simulink model "Simulink_UDP"  (R2022a)
settings: Solver=FixedStepAuto  StartTime=0.0  StopTime=100  FixedStep=0.001  RelTol=1e-3
libraries: dspnetwork x2
settings Model: Creator=dongxh  LastModifiedBy=dongxh

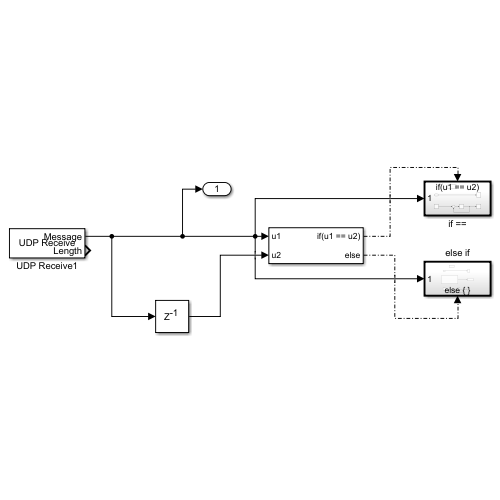
[thumbnail: Simulink's stored preview of the top-level diagram]
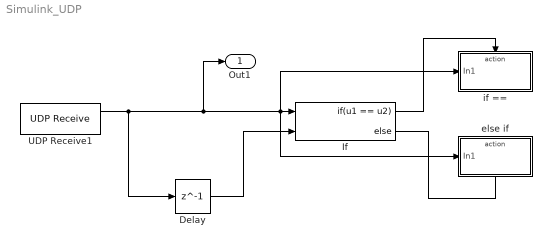
== system Simulink_UDP ==
  Delay : Delay  DelayLength=1  InitialCondition=0
  If : If  NumInputs=2  IfExpression=u1 == u2
  UDP Receive1 : dspnetwork/UDP Receive  localURL='0.0.0.0'  localPort=8002  remoteURL='127.0.0.1'  remotePort=-1  recvBufferSize=16  dims=1  signalDatatype=double  isComplex=off  isVarSize=off  showBlockingTime=off  blockingTime=0  sampletime=0.001  blockPlatform=[]
  else if : Subsystem  TreatAsAtomicUnit=on
  if == : Subsystem  TreatAsAtomicUnit=on
  Out1 : Outport
  wires:
  UDP Receive1/1 -> Delay/1, Out1/1, if ==/1(In1), If/1, else if/1(In1)
  Delay/1 -> If/2
  If/1 -> if ==/Action
  If/2 -> else if/Action

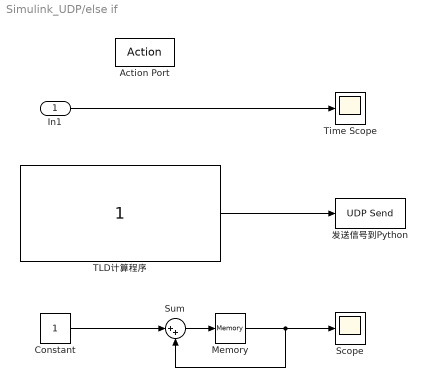
== system Simulink_UDP/else if ==
  In1 : Inport
  Action Port : ActionPort  ActionPortLabel=else
  Constant : Constant
  Memory : Memory  InheritSampleTime=on
  Scope : Scope
  Sum : Sum  Inputs=|++
  TLD计算程序 : Constant
  Time Scope : Scope
  发送信号到Python : dspnetwork/UDP Send  remoteURL='127.0.0.1'  remotePort=8004  localURL='0.0.0.0'  localPortSource=Specify via dialog  localPort=8001  sendBufferSize=16  sampletime=-1  blockPlatform=[]  separateLengthPort=0
  wires:
  Constant/1 -> Sum/1
  Sum/1 -> Memory/1
  Memory/1 -> Sum/2, Scope/1
  In1/1 -> Time Scope/1
  TLD计算程序/1 -> 发送信号到Python/1

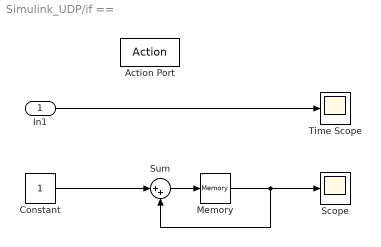
== system Simulink_UDP/if == ==
  In1 : Inport
  Action Port : ActionPort  ActionPortLabel=if(u1 == u2)
  Constant : Constant
  Memory : Memory  InheritSampleTime=on
  Scope : Scope
  Sum : Sum  Inputs=|++
  Time Scope : Scope
  wires:
  In1/1 -> Time Scope/1
  Sum/1 -> Memory/1
  Memory/1 -> Sum/2, Scope/1
  Constant/1 -> Sum/1
